simulink model "MathModel_Buck_Subsys_ClosedLoop"  (R2015a)
settings: Solver=ode45  StartTime=0.0  StopTime=0.2  RelTol=1e-3
libraries: simulink x1, powerlib_meascontrol x1
settings Model: Creator=Landon  LastModifiedBy=Landon

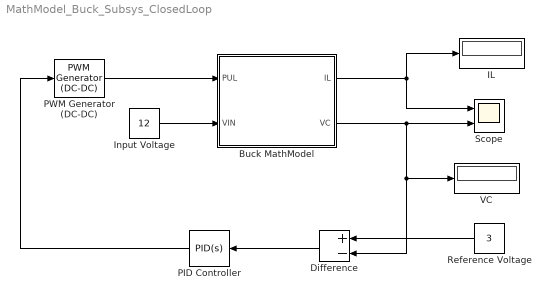
== system MathModel_Buck_Subsys_ClosedLoop ==
  Buck MathModel : Subsystem  mask{L=1.5e-3, C=250e-6, R=3}
      mask prompts: L "Inductance (H)"; C "Capacitance (F)"; R "Load Resistance (Ohm)"
  Difference : Sum  Inputs=+-
  IL : Display
  Input Voltage : Constant  Value=12
  PID Controller : simulink/Continuous/PID Controller  Controller=PID  TimeDomain=Continuous-time  SampleTime=-1  IntegratorMethod=Forward Euler  FilterMethod=Forward Euler  Form=Parallel  UseFilter=on  ControllerParametersSource=internal  P=0  I=20  D=0  N=100  InitialConditionSource=internal  InitialConditionForIntegrator=0  InitialConditionForFilter=0  ExternalReset=none  LimitOutput=off  UpperSaturationLimit=inf  LowerSaturationLimit=-inf  LinearizeAsGain=on  AntiWindupMode=none  Kb=1  TrackingMode=off  Kt=1  PParamMin=[]  PParamMax=[]  IParamMin=[]  IParamMax=[]  DParamMin=[]  DParamMax=[]  NParamMin=[]  NParamMax=[]  KbParamMin=[]  KbParamMax=[]  KtParamMin=[]  KtParamMax=[]  POutMin=[]  POutMax=[]  IOutMin=[]  IOutMax=[]  DOutMin=[]  DOutMax=[]  NOutMin=[]  NOutMax=[]  KbOutMin=[]  KbOutMax=[]  KtOutMin=[]  KtOutMax=[]  IntegratorOutMin=[]  IntegratorOutMax=[]  FilterOutMin=[]  FilterOutMax=[]  SumOutMin=[]  SumOutMax=[]  SumI1OutMin=[]  SumI1OutMax=[]  SumI2OutMin=[]  SumI2OutMax=[]  SumI3OutMin=[]  SumI3OutMax=[]  SumDOutMin=[]  SumDOutMax=[]  SaturationOutMin=[]  SaturationOutMax=[]  IntegratorContinuousStateAttributes=''  IntegratorStateMustResolveToSignalObject=off  IntegratorRTWStateStorageClass=Auto  FilterContinuousStateAttributes=''  FilterStateMustResolveToSignalObject=off  FilterRTWStateStorageClass=Auto  DifferentiatorICPrevScaledInput=0  DifferentiatorOutMin=[]  DifferentiatorOutMax=[]
  PWM Generator (DC-DC) : powerlib_meascontrol/Pulse & Signal Generators/PWM Generator (DC-DC)  Fsw=5000  Ts=0
  Reference Voltage : Constant  Value=3
  Scope : Scope  NumInputPorts=2
      settings: YMin=-5~-5  YMax=5~5
  VC : Display
  wires:
  Difference/1 -> PID Controller/1
  Reference Voltage/1 -> Difference/1
  PID Controller/1 -> PWM Generator (DC-DC)/1
  Buck MathModel/2(VC) -> Difference/2, VC/1, Scope/2
  Buck MathModel/1(IL) -> Scope/1, IL/1
  PWM Generator (DC-DC)/1 -> Buck MathModel/1(PUL)
  Input Voltage/1 -> Buck MathModel/2(VIN)

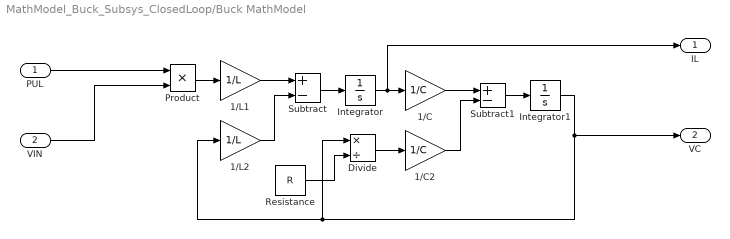
== system MathModel_Buck_Subsys_ClosedLoop/Buck MathModel ==
  PUL : Inport
  VIN : Inport  Port=2
  1/C : Gain  Gain=1/C
  1/C2 : Gain  Gain=1/C
  1/L1 : Gain  Gain=1/L
  1/L2 : Gain  Gain=1/L
  Divide : Product  Inputs=*/
  Integrator : Integrator
  Integrator1 : Integrator
  Product : Product
  Resistance : Constant  Value=R
  Subtract : Sum  Inputs=+-
  Subtract1 : Sum  Inputs=+-
  IL : Outport
  VC : Outport  Port=2
  wires:
  1/L2/1 -> Subtract/2
  1/C2/1 -> Subtract1/2
  Integrator1/1 -> 1/L2/1, Divide/1, VC/1
  Subtract/1 -> Integrator/1
  Integrator/1 -> IL/1, 1/C/1
  Resistance/1 -> Divide/2
  Subtract1/1 -> Integrator1/1
  1/L1/1 -> Subtract/1
  Product/1 -> 1/L1/1
  Divide/1 -> 1/C2/1
  1/C/1 -> Subtract1/1
  VIN/1 -> Product/2
  PUL/1 -> Product/1
